simulink model "Reference_model_PID"  (R2020b)
settings: Solver=VariableStepAuto  StartTime=0.0  StopTime=10.0  RelTol=1e-3
values from neighbouring files (symbols this model uses):
  Kd = 0.15    [dict1.sldd]
  Ki = 500.0    [dict1.sldd]
  Kp = 21.0    [dict1.sldd]
settings Model: DataDictionary=dict1.sldd  Creator=Sudhanshu  LastModifiedBy=Sudhanshu
settings DataIOCC: SaveOutput=off  SaveTime=off

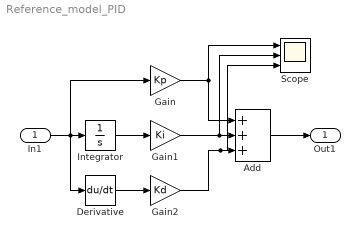
== system Reference_model_PID ==
  In1 : Inport  OutDataTypeStr=double  PortDimensions=1  SampleTime=0
  Add : Sum  Inputs=+++
  Derivative : Derivative
  Gain : Gain  Gain=Kp
  Gain1 : Gain  Gain=Ki
  Gain2 : Gain  Gain=Kd
  Integrator : Integrator
  Scope : Scope  NumInputPorts=3
  Out1 : Outport  OutDataTypeStr=double  PortDimensions=1  SampleTime=0
  wires:
  Derivative/1 -> Gain2/1
  In1/1 -> Integrator/1, Gain/1, Derivative/1
  Gain1/1 -> Scope/2, Add/2
  Add/1 -> Out1/1
  Integrator/1 -> Gain1/1
  Gain/1 -> Add/1, Scope/1
  Gain2/1 -> Scope/3, Add/3
